simulink model "zhengji"  (Simulink 8.3)
settings: Solver=ode45  StartTime=0.0  StopTime=100  RelTol=1e-3
libraries: simulink_need_slupdate x2
(part 3 of 3)

== system zhengji/GT2/LC/Subsystem3 ==
  Gz : Inport
  nz : Inport  Port=2
  Lookup Table (2-D) : Lookup2D  RowIndex=[4300 5000 5500 6000 6500 7000 7500 8000]  ColumnIndex=[20:0.5:100]  Table=|
      | [1.1111 1.1471 1.1832 1.2192 1.2552 1.2913 1.3273 1.3633 1.3994 1.4354 1.4714 1.5074 1.5435 1.5795 1.6155 1.6516 1.6876 1.7236 1.8750 1.8749 1.8720 1.8623 1.8457 1.8223 1.7920 1.7549 1.7109 1.6601 1.6024 1.5378 1.4664 1.3881 1.2420 1.2701 1.2983 1.3265 1.3547 1.3828 1.4110 1.4392 1.4673 1.4955 1.5237 1.5519 1.5800 1.6082 1.6364 1.6645 1.6927 1.7209 1.7491 1.7772 1.8054 1.8336 1.8617 1.8899 1.9181 1.9463 1.9744 2.0026 2.0308 2.0590 2.0871 2.1153 2.1435 2.1716 2.1998 2.2280 2.2562 2.2843 2.3125 2.3407 2.3688 2.3970 2.4252 2.4534 2.4815 2.5097 2.5379 2.5660 2.5942 2.6224 2.6506 2.6787 2.7069 2.7351 2.7633 2.7914 2.8196 2.8478 2.8759 2.9041 2.9323 2.9605 2.9886 3.0168 3.0450 3.0731 3.1013 3.1295 3.1577 3.1858 3.2140 3.2422 3.2703 3.2985 3.3267 3.3549 3.3830 3.4112 3.4394 3.4676 3.4957 3.5239 3.5521 3.5802 3.6084 3.6366 3.6648 3.6929 3.7211 3.7493 3.7774 3.8056 3.8338 3.8620 3.8901 3.9183 3.9465 3.9746 4.0028 4.0310 4.0592 4.0873 4.1155 4.1437 4.1719 4.2000 4.2282 4.2564 4.2845 4.3127 4.3409 4.3691 4.3972 4.4254 4.4536 4.4817 4.5099 4.5381 4.5663 4.5944 4.6226 4.6508 4.6789 4.7071 4.7353 4.7635 4.7916 4.8198 4.8480;
      | 1.1111 1.1471 1.1832 1.2192 1.2552 1.2913 1.3273 1.3633 1.3994 1.4354 1.4714 1.5074 1.5435 1.5795 1.6155 1.6516 1.6876 1.7236 1.7597 1.7957 1.8317 1.8678 1.9038 1.9398 1.9758 2.0119 2.0479 2.0839 2.1200 2.1560 2.1920 2.2281 2.2641 2.3001 2.3361 2.3722 2.4082 2.4442 2.4803 2.5163 2.5523 2.5884 2.5200 2.4780 2.3700 2.2800 2.1500 1.8820 1.6080 1.7209 1.7491 1.7772 1.8054 1.8336 1.8617 1.8899 1.9181 1.9463 1.9744 2.0026 2.0308 2.0590 2.0871 2.1153 2.1435 2.1716 2.1998 2.2280 2.2562 2.2843 2.3125 2.3407 2.3688 2.3970 2.4252 2.4534 2.4815 2.5097 2.5379 2.5660 2.5942 2.6224 2.6506 2.6787 2.7069 2.7351 2.7633 2.7914 2.8196 2.8478 2.8759 2.9041 2.9323 2.9605 2.9886 3.0168 3.0450 3.0731 3.1013 3.1295 3.1577 3.1858 3.2140 3.2422 3.2703 3.2985 3.3267 3.3549 3.3830 3.4112 3.4394 3.4676 3.4957 3.5239 3.5521 3.5802 3.6084 3.6366 3.6648 3.6929 3.7211 3.7493 3.7774 3.8056 3.8338 3.8620 3.8901 3.9183 3.9465 3.9746 4.0028 4.0310 4.0592 4.0873 4.1155 4.1437 4.1719 4.2000 4.2282 4.2564 4.2845 4.3127 4.3409 4.3691 4.3972 4.4254 4.4536 4.4817 4.5099 4.5381 4.5663 4.5944 4.6226 4.6508 4.6789 4.7071 4.7353 4.7635 4.7916 4.8198 4.8480;
      | 1.1111 1.1471 1.1832 1.2192 1.2552 1.2913 1.3273 1.3633 1.3994 1.4354 1.4714 1.5074 1.5435 1.5795 1.6155 1.6516 1.6876 1.7236 1.7597 1.7957 1.8317 1.8678 1.9038 1.9398 1.9758 2.0119 2.0479 2.0839 2.1200 2.1560 2.1920 2.2281 2.2641 2.3001 2.3361 2.3722 2.4082 2.4442 2.4803 2.5163 2.5523 2.5884 2.6244 2.6604 2.6965 2.7325 2.7685 2.8045 2.8406 2.8766 2.9126 2.9487 2.9847 3.0207 2.8905 2.8292 2.7444 2.6661 2.5443 2.4489 2.3700 2.1776 2.0217 2.1153 2.1435 2.1716 2.1998 2.2280 2.2562 2.2843 2.3125 2.3407 2.3688 2.3970 2.4252 2.4534 2.4815 2.5097 2.5379 2.5660 2.5942 2.6224 2.6506 2.6787 2.7069 2.7351 2.7633 2.7914 2.8196 2.8478 2.8759 2.9041 2.9323 2.9605 2.9886 3.0168 3.0450 3.0731 3.1013 3.1295 3.1577 3.1858 3.2140 3.2422 3.2703 3.2985 3.3267 3.3549 3.3830 3.4112 3.4394 3.4676 3.4957 3.5239 3.5521 3.5802 3.6084 3.6366 3.6648 3.6929 3.7211 3.7493 3.7774 3.8056 3.8338 3.8620 3.8901 3.9183 3.9465 3.9746 4.0028 4.0310 4.0592 4.0873 4.1155 4.1437 4.1719 4.2000 4.2282 4.2564 4.2845 4.3127 4.3409 4.3691 4.3972 4.4254 4.4536 4.4817 4.5099 4.5381 4.5663 4.5944 4.6226 4.6508 4.6789 4.7071 4.7353 4.7635 4.7916 4.8198 4.8480;
      | 1.1111 1.1471 1.1832 1.2192 1.2552 1.2913 1.3273 1.3633 1.3994 1.4354 1.4714 1.5074 1.5435 1.5795 1.6155 1.6516 1.6876 1.7236 1.7597 1.7957 1.8317 1.8678 1.9038 1.9398 1.9758 2.0119 2.0479 2.0839 2.1200 2.1560 2.1920 2.2281 2.2641 2.3001 2.3361 2.3722 2.4082 2.4442 2.4803 2.5163 2.5523 2.5884 2.6244 2.6604 2.6965 2.7325 2.7685 2.8045 2.8406 2.8766 2.9126 2.9487 2.9847 3.0207 3.0568 3.0928 3.1288 3.1648 3.2009 3.2369 3.2729 3.3090 3.3450 3.3810 3.3655 3.3396 3.3040 3.2587 3.2037 3.1389 3.0645 2.9803 2.8865 2.7829 2.6696 2.5466 2.4815 2.5097 2.5379 2.5660 2.5942 2.6224 2.6506 2.6787 2.7069 2.7351 2.7633 2.7914 2.8196 2.8478 2.8759 2.9041 2.9323 2.9605 2.9886 3.0168 3.0450 3.0731 3.1013 3.1295 3.1577 3.1858 3.2140 3.2422 3.2703 3.2985 3.3267 3.3549 3.3830 3.4112 3.4394 3.4676 3.4957 3.5239 3.5521 3.5802 3.6084 3.6366 3.6648 3.6929 3.7211 3.7493 3.7774 3.8056 3.8338 3.8620 3.8901 3.9183 3.9465 3.9746 4.0028 4.0310 4.0592 4.0873 4.1155 4.1437 4.1719 4.2000 4.2282 4.2564 4.2845 4.3127 4.3409 4.3691 4.3972 4.4254 4.4536 4.4817 4.5099 4.5381 4.5663 4.5944 4.6226 4.6508 4.6789 4.7071 4.7353 4.7635 4.7916 4.8198 4.8480;
      | 1.1111 1.1471 1.1832 1.2192 1.2552 1.2913 1.3273 1.3633 1.3994 1.4354 1.4714 1.5074 1.5435 1.5795 1.6155 1.6516 1.6876 1.7236 1.7597 1.7957 1.8317 1.8678 1.9038 1.9398 1.9758 2.0119 2.0479 2.0839 2.1200 2.1560 2.1920 2.2281 2.2641 2.3001 2.3361 2.3722 2.4082 2.4442 2.4803 2.5163 2.5523 2.5884 2.6244 2.6604 2.6965 2.7325 2.7685 2.8045 2.8406 2.8766 2.9126 2.9487 2.9847 3.0207 3.0568 3.0928 3.1288 3.1648 3.2009 3.2369 3.2729 3.3090 3.3450 3.3810 3.4171 3.4531 3.4891 3.5252 3.5612 3.5972 3.6332 3.6693 3.7053 3.7413 3.7774 3.8134 3.8494 3.8855 3.9215 3.9575 3.9936 4.0296 4.0656 4.1016 4.1377 4.1737 4.2097 4.2458 4.2818 4.3178 4.3646 4.3478 4.3218 4.2866 4.2421 4.1884 4.1254 4.0533 3.9718 3.8812 3.7813 3.6722 3.5538 3.4262 3.2894 3.2985 3.3267 3.3549 3.3830 3.4112 3.4394 3.4676 3.4957 3.5239 3.5521 3.5802 3.6084 3.6366 3.6648 3.6929 3.7211 3.7493 3.7774 3.8056 3.8338 3.8620 3.8901 3.9183 3.9465 3.9746 4.0028 4.0310 4.0592 4.0873 4.1155 4.1437 4.1719 4.2000 4.2282 4.2564 4.2845 4.3127 4.3409 4.3691 4.3972 4.4254 4.4536 4.4817 4.5099 4.5381 4.5663 4.5944 4.6226 4.6508 4.6789 4.7071 4.7353 4.7635 4.7916 4.8198 4.8480;
      | 1.1111 1.1471 1.1832 1.2192 1.2552 1.2913 1.3273 1.3633 1.3994 1.4354 1.4714 1.5074 1.5435 1.5795 1.6155 1.6516 1.6876 1.7236 1.7597 1.7957 1.8317 1.8678 1.9038 1.9398 1.9758 2.0119 2.0479 2.0839 2.1200 2.1560 2.1920 2.2281 2.2641 2.3001 2.3361 2.3722 2.4082 2.4442 2.4803 2.5163 2.5523 2.5884 2.6244 2.6604 2.6965 2.7325 2.7685 2.8045 2.8406 2.8766 2.9126 2.9487 2.9847 3.0207 3.0568 3.0928 3.1288 3.1648 3.2009 3.2369 3.2729 3.3090 3.3450 3.3810 3.4171 3.4531 3.4891 3.5252 3.5612 3.5972 3.6332 3.6693 3.7053 3.7413 3.7774 3.8134 3.8494 3.8855 3.9215 3.9575 3.9936 4.0296 4.0656 4.1016 4.1377 4.1737 4.2097 4.2458 4.2818 4.3178 4.3539 4.3899 4.4259 4.4619 4.4980 4.5340 4.5700 4.6061 4.6421 4.6781 4.7142 4.7502 4.7862 4.8223 4.8583 4.8943 4.9303 4.9664 5.0024 5.0384 5.0745 5.1105 5.1465 5.3241 5.3091 5.2474 5.1391 4.9841 4.7824 4.5341 4.2392 3.8976 3.7774 3.8056 3.8338 3.8620 3.8901 3.9183 3.9465 3.9746 4.0028 4.0310 4.0592 4.0873 4.1155 4.1437 4.1719 4.2000 4.2282 4.2564 4.2845 4.3127 4.3409 4.3691 4.3972 4.4254 4.4536 4.4817 4.5099 4.5381 4.5663 4.5944 4.6226 4.6508 4.6789 4.7071 4.7353 4.7635 4.7916 4.8198 4.8480;
      | 1.1111 1.1471 1.1832 1.2192 1.2552 1.2913 1.3273 1.3633 1.3994 1.4354 1.4714 1.5074 1.5435 1.5795 1.6155 1.6516 1.6876 1.7236 1.7597 1.7957 1.8317 1.8678 1.9038 1.9398 1.9758 2.0119 2.0479 2.0839 2.1200 2.1560 2.1920 2.2281 2.2641 2.3001 2.3361 2.3722 2.4082 2.4442 2.4803 2.5163 2.5523 2.5884 2.6244 2.6604 2.6965 2.7325 2.7685 2.8045 2.8406 2.8766 2.9126 2.9487 2.9847 3.0207 3.0568 3.0928 3.1288 3.1648 3.2009 3.2369 3.2729 3.3090 3.3450 3.3810 3.4171 3.4531 3.4891 3.5252 3.5612 3.5972 3.6332 3.6693 3.7053 3.7413 3.7774 3.8134 3.8494 3.8855 3.9215 3.9575 3.9936 4.0296 4.0656 4.1016 4.1377 4.1737 4.2097 4.2458 4.2818 4.3178 4.3539 4.3899 4.4259 4.4619 4.4980 4.5340 4.5700 4.6061 4.6421 4.6781 4.7142 4.7502 4.7862 4.8223 4.8583 4.8943 4.9303 4.9664 5.0024 5.0384 5.0745 5.1105 5.1465 5.1826 5.2186 5.2546 5.2906 5.3267 5.3627 5.3987 5.4348 5.4708 5.5068 5.5429 5.5789 5.6149 5.6510 5.6870 5.7230 5.7590 5.7951 5.8311 5.8671 5.9032 5.9392 5.9752 6.0113 6.0473 5.2600 4.2400 4.2845 4.3127 4.3409 4.3691 4.3972 4.4254 4.4536 4.4817 4.5099 4.5381 4.5663 4.5944 4.6226 4.6508 4.6789 4.7071 4.7353 4.7635 4.7916 4.8198 4.8480;
      | 1.1111 1.1471 1.1832 1.2192 1.2552 1.2913 1.3273 1.3633 1.3994 1.4354 1.4714 1.5074 1.5435 1.5795 1.6155 1.6516 1.6876 1.7236 1.7597 1.7957 1.8317 1.8678 1.9038 1.9398 1.9758 2.0119 2.0479 2.0839 2.1200 2.1560 2.1920 2.2281 2.2641 2.3001 2.3361 2.3722 2.4082 2.4442 2.4803 2.5163 2.5523 2.5884 2.6244 2.6604 2.6965 2.7325 2.7685 2.8045 2.8406 2.8766 2.9126 2.9487 2.9847 3.0207 3.0568 3.0928 3.1288 3.1648 3.2009 3.2369 3.2729 3.3090 3.3450 3.3810 3.4171 3.4531 3.4891 3.5252 3.5612 3.5972 3.6332 3.6693 3.7053 3.7413 3.7774 3.8134 3.8494 3.8855 3.9215 3.9575 3.9936 4.0296 4.0656 4.1016 4.1377 4.1737 4.2097 4.2458 4.2818 4.3178 4.3539 4.3899 4.4259 4.4619 4.4980 4.5340 4.5700 4.6061 4.6421 4.6781 4.7142 4.7502 4.7862 4.8223 4.8583 4.8943 4.9303 4.9664 5.0024 5.0384 5.0745 5.1105 5.1465 5.1826 5.2186 5.2546 5.2906 5.3267 5.3627 5.3987 5.4348 5.4708 5.5068 5.5429 5.5789 5.6149 5.6510 5.6870 5.7230 5.7590 5.7951 5.8311 5.8671 5.9032 5.9392 5.9752 6.0113 6.0473 6.0833 6.1193 6.1554 6.1914 6.2274 6.2635 6.2995 6.3355 6.3716 6.4076 6.4436 6.4797 6.5157 6.5517 6.5877 6.6238 6.6598 4.7071 4.7353 4.7635 4.7916 4.8198 4.8480;]
  Lookup Table (2-D)1 : Lookup2D  RowIndex=[4300 5000 5500 6000 6500 7000 7500 8000]  ColumnIndex=[20:0.5:100]  Table=|
      | [0.8303 0.8307 0.8310 0.8314 0.8317 0.8321 0.8324 0.8327 0.8331 0.8335 0.8338 0.8341 0.8345 0.8348 0.8351 0.8355 0.8358 0.8361 0.8371 0.8390 0.8403 0.8412 0.8415 0.8412 0.8405 0.8392 0.8373 0.8350 0.8321 0.8287 0.8247 0.8203 0.8200 0.8200 0.8200 0.8200 0.8200 0.8200 0.8200 0.8200 0.8200 0.8200 0.8200 0.8200 0.8200 0.8200 0.8200 0.8200 0.8200 0.8200 0.8200 0.8200 0.8200 0.8200 0.8200 0.8200 0.8200 0.8200 0.8200 0.8200 0.8200 0.8200 0.8200 0.8200 0.8200 0.8200 0.8200 0.8200 0.8200 0.8200 0.8200 0.8200 0.8200 0.8200 0.8200 0.8200 0.8200 0.8200 0.8200 0.8200 0.8200 0.8200 0.8200 0.8200 0.8200 0.8200 0.8200 0.8200 0.8200 0.8200 0.8200 0.8200 0.8200 0.8200 0.8200 0.8200 0.8200 0.8200 0.8200 0.8200 0.8200 0.8200 0.8200 0.8200 0.8200 0.8500 0.8500 0.8500 0.8500 0.8500 0.8500 0.8500 0.8500 0.8500 0.8500 0.8500 0.8500 0.8500 0.8500 0.8500 0.8500 0.8500 0.8500 0.8500 0.8500 0.8500 0.8500 0.8500 0.8500 0.8500 0.8500 0.8500 0.8500 0.8500 0.8500 0.8500 0.8500 0.8500 0.8500 0.8500 0.8500 0.8500 0.8500 0.8500 0.8500 0.8500 0.8500 0.8500 0.8500 0.8500 0.8500 0.8500 0.8500 0.8500 0.8500 0.8500 0.8500 0.8500 0.8500 0.8500 0.8500;
      | 0.8303 0.8307 0.8310 0.8314 0.8317 0.8321 0.8324 0.8327 0.8331 0.8335 0.8338 0.8341 0.8345 0.8348 0.8351 0.8355 0.8358 0.8361 0.8371 0.8375 0.8379 0.8383 0.8387 0.8391 0.8395 0.8400 0.8402 0.8405 0.8407 0.8410 0.8412 0.8415 0.8417 0.8420 0.8422 0.8425 0.8427 0.8430 0.8432 0.8435 0.8437 0.8440 0.8441 0.8727 0.8851 0.8814 0.8616 0.8257 0.8200 0.8200 0.8200 0.8200 0.8200 0.8200 0.8200 0.8200 0.8200 0.8200 0.8200 0.8200 0.8200 0.8200 0.8200 0.8200 0.8200 0.8200 0.8200 0.8200 0.8200 0.8200 0.8200 0.8200 0.8200 0.8200 0.8200 0.8200 0.8200 0.8200 0.8200 0.8200 0.8200 0.8200 0.8200 0.8200 0.8200 0.8200 0.8200 0.8200 0.8200 0.8200 0.8200 0.8200 0.8200 0.8200 0.8200 0.8200 0.8200 0.8200 0.8200 0.8200 0.8200 0.8200 0.8200 0.8200 0.8200 0.8500 0.8500 0.8500 0.8500 0.8500 0.8500 0.8500 0.8500 0.8500 0.8500 0.8500 0.8500 0.8500 0.8500 0.8500 0.8500 0.8500 0.8500 0.8500 0.8500 0.8500 0.8500 0.8500 0.8500 0.8500 0.8500 0.8500 0.8500 0.8500 0.8500 0.8500 0.8500 0.8500 0.8500 0.8500 0.8500 0.8500 0.8500 0.8500 0.8500 0.8500 0.8500 0.8500 0.8500 0.8500 0.8500 0.8500 0.8500 0.8500 0.8500 0.8500 0.8500 0.8500 0.8500 0.8500 0.8500;
      | 0.8303 0.8307 0.8310 0.8314 0.8317 0.8321 0.8324 0.8327 0.8331 0.8335 0.8338 0.8341 0.8345 0.8348 0.8351 0.8355 0.8358 0.8361 0.8371 0.8375 0.8379 0.8383 0.8387 0.8391 0.8395 0.8400 0.8402 0.8405 0.8407 0.8410 0.8412 0.8415 0.8417 0.8420 0.8422 0.8425 0.8427 0.8430 0.8432 0.8435 0.8437 0.8440 0.8441 0.8440 0.8440 0.8440 0.8440 0.8440 0.8400 0.8400 0.8400 0.8400 0.8400 0.8400 0.8400 0.8400 0.8420 0.8439 0.8592 0.8652 0.8619 0.8495 0.8278 0.8200 0.8200 0.8200 0.8200 0.8200 0.8200 0.8200 0.8200 0.8200 0.8200 0.8200 0.8200 0.8200 0.8200 0.8200 0.8200 0.8200 0.8200 0.8200 0.8200 0.8200 0.8200 0.8200 0.8200 0.8200 0.8200 0.8200 0.8200 0.8200 0.8200 0.8200 0.8200 0.8200 0.8200 0.8200 0.8200 0.8200 0.8200 0.8200 0.8200 0.8200 0.8200 0.8500 0.8500 0.8500 0.8500 0.8500 0.8500 0.8500 0.8500 0.8500 0.8500 0.8500 0.8500 0.8500 0.8500 0.8500 0.8500 0.8500 0.8500 0.8500 0.8500 0.8500 0.8500 0.8500 0.8500 0.8500 0.8500 0.8500 0.8500 0.8500 0.8500 0.8500 0.8500 0.8500 0.8500 0.8500 0.8500 0.8500 0.8500 0.8500 0.8500 0.8500 0.8500 0.8500 0.8500 0.8500 0.8500 0.8500 0.8500 0.8500 0.8500 0.8500 0.8500 0.8500 0.8500 0.8500 0.8500;
      | 0.8303 0.8307 0.8310 0.8314 0.8317 0.8321 0.8324 0.8327 0.8331 0.8335 0.8338 0.8341 0.8345 0.8348 0.8351 0.8355 0.8358 0.8361 0.8371 0.8375 0.8379 0.8383 0.8387 0.8391 0.8395 0.8400 0.8402 0.8405 0.8407 0.8410 0.8412 0.8415 0.8417 0.8420 0.8422 0.8425 0.8427 0.8430 0.8432 0.8435 0.8437 0.8440 0.8441 0.8440 0.8440 0.8440 0.8440 0.8440 0.8400 0.8400 0.8400 0.8400 0.8400 0.8400 0.8400 0.8390 0.8380 0.8370 0.8360 0.8350 0.8340 0.8330 0.8320 0.8310 0.8300 0.8300 0.8300 0.8371 0.8489 0.8568 0.8608 0.8609 0.8570 0.8492 0.8375 0.8219 0.8200 0.8200 0.8200 0.8200 0.8200 0.8200 0.8200 0.8200 0.8200 0.8200 0.8200 0.8200 0.8200 0.8200 0.8200 0.8200 0.8200 0.8200 0.8200 0.8200 0.8200 0.8200 0.8200 0.8200 0.8200 0.8200 0.8200 0.8200 0.8200 0.8500 0.8500 0.8500 0.8500 0.8500 0.8500 0.8500 0.8500 0.8500 0.8500 0.8500 0.8500 0.8500 0.8500 0.8500 0.8500 0.8500 0.8500 0.8500 0.8500 0.8500 0.8500 0.8500 0.8500 0.8500 0.8500 0.8500 0.8500 0.8500 0.8500 0.8500 0.8500 0.8500 0.8500 0.8500 0.8500 0.8500 0.8500 0.8500 0.8500 0.8500 0.8500 0.8500 0.8500 0.8500 0.8500 0.8500 0.8500 0.8500 0.8500 0.8500 0.8500 0.8500 0.8500 0.8500 0.8500;
      | 0.8303 0.8307 0.8310 0.8314 0.8317 0.8321 0.8324 0.8327 0.8331 0.8335 0.8338 0.8341 0.8345 0.8348 0.8351 0.8355 0.8358 0.8361 0.8371 0.8375 0.8379 0.8383 0.8387 0.8391 0.8395 0.8400 0.8402 0.8405 0.8407 0.8410 0.8412 0.8415 0.8417 0.8420 0.8422 0.8425 0.8427 0.8430 0.8432 0.8435 0.8437 0.8440 0.8441 0.8440 0.8440 0.8440 0.8440 0.8440 0.8400 0.8400 0.8400 0.8400 0.8400 0.8400 0.8400 0.8390 0.8380 0.8370 0.8360 0.8350 0.8340 0.8330 0.8320 0.8310 0.8300 0.8306 0.8312 0.8318 0.8324 0.8330 0.8336 0.8342 0.8348 0.8354 0.8360 0.8366 0.8372 0.8378 0.8384 0.8390 0.8396 0.8402 0.8408 0.8414 0.8420 0.8426 0.8432 0.8435 0.8438 0.8442 0.8438 0.8515 0.8581 0.8636 0.8680 0.8712 0.8733 0.8743 0.8742 0.8730 0.8706 0.8671 0.8625 0.8568 0.8500 0.8500 0.8500 0.8500 0.8500 0.8500 0.8500 0.8500 0.8500 0.8500 0.8500 0.8500 0.8500 0.8500 0.8500 0.8500 0.8500 0.8500 0.8500 0.8500 0.8500 0.8500 0.8500 0.8500 0.8500 0.8500 0.8500 0.8500 0.8500 0.8500 0.8500 0.8500 0.8500 0.8500 0.8500 0.8500 0.8500 0.8500 0.8500 0.8500 0.8500 0.8500 0.8500 0.8500 0.8500 0.8500 0.8500 0.8500 0.8500 0.8500 0.8500 0.8500 0.8500 0.8500 0.8500 0.8500 0.8500;
      | 0.8303 0.8307 0.8310 0.8314 0.8317 0.8321 0.8324 0.8327 0.8331 0.8335 0.8338 0.8341 0.8345 0.8348 0.8351 0.8355 0.8358 0.8361 0.8371 0.8375 0.8379 0.8383 0.8387 0.8391 0.8395 0.8400 0.8402 0.8405 0.8407 0.8410 0.8412 0.8415 0.8417 0.8420 0.8422 0.8425 0.8427 0.8430 0.8432 0.8435 0.8437 0.8440 0.8441 0.8440 0.8440 0.8440 0.8440 0.8440 0.8400 0.8400 0.8400 0.8400 0.8400 0.8400 0.8400 0.8390 0.8380 0.8370 0.8360 0.8350 0.8340 0.8330 0.8320 0.8310 0.8300 0.8306 0.8312 0.8318 0.8324 0.8330 0.8336 0.8342 0.8348 0.8354 0.8360 0.8366 0.8372 0.8378 0.8384 0.8390 0.8396 0.8402 0.8408 0.8414 0.8420 0.8426 0.8432 0.8435 0.8438 0.8442 0.8448 0.8452 0.8457 0.8462 0.8467 0.8472 0.8476 0.8451 0.8486 0.8491 0.8496 0.8500 0.8505 0.8510 0.8515 0.8520 0.8524 0.8529 0.8534 0.8539 0.8544 0.8548 0.8549 0.8550 0.8600 0.8650 0.8746 0.8872 0.8921 0.8890 0.8782 0.8595 0.8500 0.8500 0.8500 0.8500 0.8500 0.8500 0.8500 0.8500 0.8500 0.8500 0.8500 0.8500 0.8500 0.8500 0.8500 0.8500 0.8500 0.8500 0.8500 0.8500 0.8500 0.8500 0.8500 0.8500 0.8500 0.8500 0.8500 0.8500 0.8500 0.8500 0.8500 0.8500 0.8500 0.8500 0.8500 0.8500 0.8500 0.8500 0.8500;
      | 0.8303 0.8307 0.8310 0.8314 0.8317 0.8321 0.8324 0.8327 0.8331 0.8335 0.8338 0.8341 0.8345 0.8348 0.8351 0.8355 0.8358 0.8361 0.8371 0.8375 0.8379 0.8383 0.8387 0.8391 0.8395 0.8400 0.8402 0.8405 0.8407 0.8410 0.8412 0.8415 0.8417 0.8420 0.8422 0.8425 0.8427 0.8430 0.8432 0.8435 0.8437 0.8440 0.8441 0.8440 0.8440 0.8440 0.8440 0.8440 0.8400 0.8400 0.8400 0.8400 0.8400 0.8400 0.8400 0.8390 0.8380 0.8370 0.8360 0.8350 0.8340 0.8330 0.8320 0.8310 0.8300 0.8306 0.8312 0.8318 0.8324 0.8330 0.8336 0.8342 0.8348 0.8354 0.8360 0.8366 0.8372 0.8378 0.8384 0.8390 0.8396 0.8402 0.8408 0.8414 0.8420 0.8426 0.8432 0.8435 0.8438 0.8442 0.8448 0.8452 0.8457 0.8462 0.8467 0.8472 0.8476 0.8451 0.8486 0.8491 0.8496 0.8500 0.8505 0.8510 0.8515 0.8520 0.8524 0.8529 0.8534 0.8539 0.8544 0.8548 0.8549 0.8550 0.8550 0.8550 0.8550 0.8550 0.8550 0.8550 0.8550 0.8550 0.8550 0.8550 0.8550 0.8550 0.8550 0.8550 0.8550 0.8550 0.8550 0.8550 0.8550 0.8550 0.8550 0.8550 0.8550 0.8550 0.8788 0.8500 0.8500 0.8500 0.8500 0.8500 0.8500 0.8500 0.8500 0.8500 0.8500 0.8500 0.8500 0.8500 0.8500 0.8500 0.8500 0.8500 0.8500 0.8500 0.8500 0.8500 0.8500;
      | 0.8303 0.8307 0.8310 0.8314 0.8317 0.8321 0.8324 0.8327 0.8331 0.8335 0.8338 0.8341 0.8345 0.8348 0.8351 0.8355 0.8358 0.8361 0.8371 0.8375 0.8379 0.8383 0.8387 0.8391 0.8395 0.8400 0.8402 0.8405 0.8407 0.8410 0.8412 0.8415 0.8417 0.8420 0.8422 0.8425 0.8427 0.8430 0.8432 0.8435 0.8437 0.8440 0.8441 0.8440 0.8440 0.8440 0.8440 0.8440 0.8400 0.8400 0.8400 0.8400 0.8400 0.8400 0.8400 0.8390 0.8380 0.8370 0.8360 0.8350 0.8340 0.8330 0.8320 0.8310 0.8300 0.8306 0.8312 0.8318 0.8324 0.8330 0.8336 0.8342 0.8348 0.8354 0.8360 0.8366 0.8372 0.8378 0.8384 0.8390 0.8396 0.8402 0.8408 0.8414 0.8420 0.8426 0.8432 0.8435 0.8438 0.8442 0.8448 0.8452 0.8457 0.8462 0.8467 0.8472 0.8476 0.8451 0.8486 0.8491 0.8496 0.8500 0.8505 0.8510 0.8515 0.8520 0.8524 0.8529 0.8534 0.8539 0.8544 0.8548 0.8549 0.8550 0.8550 0.8550 0.8550 0.8550 0.8550 0.8550 0.8550 0.8550 0.8550 0.8550 0.8550 0.8550 0.8550 0.8550 0.8550 0.8550 0.8550 0.8550 0.8550 0.8550 0.8550 0.8550 0.8550 0.8550 0.8550 0.8550 0.8550 0.8550 0.8550 0.8550 0.8550 0.8550 0.8550 0.8550 0.8550 0.8550 0.8550 0.8550 0.8550 0.8550 0.8550 0.8550 0.8500 0.8500 0.8500 0.8500 0.8550;]
  pi : Outport
  eta : Outport  Port=2
  wires:
  nz/1 -> Lookup Table (2-D)/1, Lookup Table (2-D)1/1
  Gz/1 -> Lookup Table (2-D)1/2, Lookup Table (2-D)/2
  Lookup Table (2-D)/1 -> pi/1
  Lookup Table (2-D)1/1 -> eta/1

== system zhengji/GT2/LC/compresser_TN ==
  Gin : Inport
  Pi : Inport  Port=2
  eta : Inport  Port=3
  Tin : Inport  Port=4
  Add : Sum  Inputs=+-
  Add1 : Sum
  Constant : Constant
  Divide : Product  Inputs=/*
  Fcn : Fcn  Expr=u[1]^(u[2])
  K : Subsystem
  K1 : Constant  Value=1.4
  Mux : Mux  Inputs=2
  Product : Product  Inputs=4  RndMeth=Zero
  Product1 : Product  RndMeth=Zero
  m : Fcn  Expr=(u-1)/u
  Tout : Outport
  Nout : Outport  Port=2
  wires:
  Tin/1 -> K/1(T1), Product1/2, Product/4
  Pi/1 -> Mux/1
  m/1 -> Mux/2
  Mux/1 -> Fcn/1
  Fcn/1 -> Add/1
  Add/1 -> Divide/2
  eta/1 -> Divide/1
  Divide/1 -> Add1/1, Product/1
  Constant/1 -> Add/2, Add1/2
  Product1/1 -> Tout/1
  Product/1 -> Nout/1
  Add1/1 -> Product1/1
  K/2(Cp) -> Product/2
  Gin/1 -> Product/3
  K1/1 -> m/1

== system zhengji/GT2/LC/zhehe ==
  n : Inport
  Tin : Inport  Port=2
  Divide : Product  Inputs=*/
  Fcn : Fcn  Expr=sqrt(u/288)
  nz : Outport
  wires:
  Tin/1 -> Fcn/1
  n/1 -> Divide/1
  Fcn/1 -> Divide/2
  Divide/1 -> nz/1

== system zhengji/GT2/LT/turbine_TN ==
  Pi : Inport
  eta : Inport  Port=2
  Tin : Inport  Port=3
  Gin : Inport  Port=4
  Add : Sum  Inputs=-+
  Add1 : Sum  Inputs=-+
  Constant : Constant
  Fcn : Fcn  Expr=1/(u[1]^u[2])
  K : Subsystem
  K1 : Constant  Value=1.33
  Mux : Mux  Inputs=2
  Product : Product  Inputs=4  RndMeth=Zero
  Product1 : Product  RndMeth=Zero
  Product2 : Product  RndMeth=Zero
  m : Fcn  Expr=(u-1)/u
  Tout : Outport
  Nout : Outport  Port=2
  wires:
  Tin/1 -> K/1(T1), Product1/2, Product/4
  Pi/1 -> Mux/1
  m/1 -> Mux/2
  Mux/1 -> Fcn/1
  Fcn/1 -> Add/1
  Add/1 -> Product2/2
  eta/1 -> Product2/1
  Product2/1 -> Add1/1, Product/1
  Constant/1 -> Add/2, Add1/2
  Product1/1 -> Tout/1
  Product/1 -> Nout/1
  Add1/1 -> Product1/1
  K/2(Cp) -> Product/2
  Gin/1 -> Product/3
  K1/1 -> m/1

== system zhengji/GT2/PT/turbine_TN ==
  Pi : Inport
  eta : Inport  Port=2
  Gin : Inport  Port=3
  Tin : Inport  Port=4
  Add : Sum  Inputs=-+
  Add1 : Sum  Inputs=-+
  Constant : Constant
  Fcn : Fcn  Expr=1/(u[1]^u[2])
  K1 : Subsystem
  Mux : Mux  Inputs=2
  Product : Product  Inputs=4  RndMeth=Zero
  Product1 : Product  RndMeth=Zero
  Product2 : Product  RndMeth=Zero
  m : Fcn  Expr=(u-1)/u
  Tout : Outport
  Nout : Outport  Port=2
  wires:
  Pi/1 -> Mux/1
  m/1 -> Mux/2
  Mux/1 -> Fcn/1
  Fcn/1 -> Add/1
  Add/1 -> Product2/2
  eta/1 -> Product2/1
  Product2/1 -> Add1/1, Product/1
  Constant/1 -> Add/2, Add1/2
  Product1/1 -> Tout/1
  Product/1 -> Nout/1
  Add1/1 -> Product1/1
  Gin/1 -> Product/3
  Tin/1 -> K1/1(T1), Product1/2, Product/4
  K1/2(Cp) -> Product/2
  K1/1(K) -> m/1

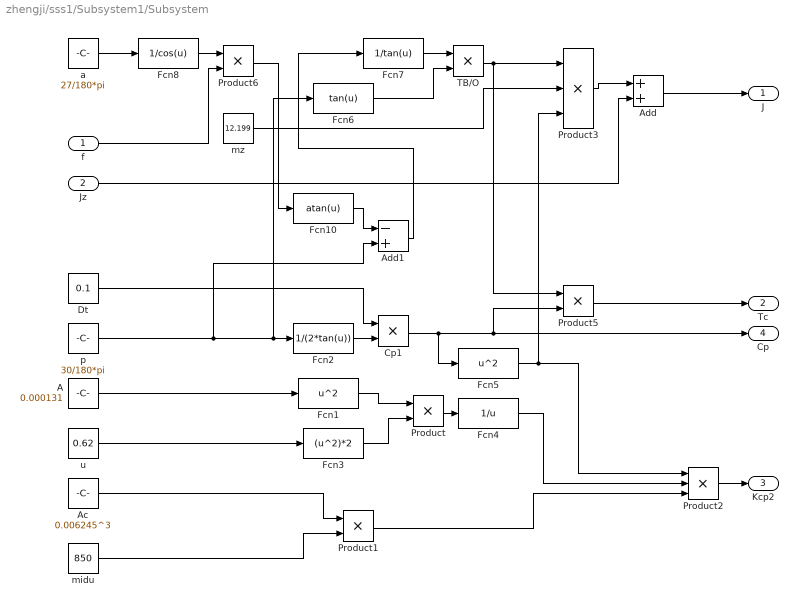
== system zhengji/sss1/Subsystem1/Subsystem ==
  f : Inport
  Jz : Inport  Port=2
  A : Constant  Value=0.000131
  Ac : Constant  Value=0.006245^3
  Add : Sum
  Add1 : Sum  Inputs=-+
  Cp1 : Product  RndMeth=Zero
  Dt : Constant  Value=0.1
  Fcn1 : Fcn  Expr=u^2
  Fcn10 : Fcn  Expr=atan(u)
  Fcn2 : Fcn  Expr=1/(2*tan(u))
  Fcn3 : Fcn  Expr=(u^2)*2
  Fcn4 : Fcn  Expr=1/u
  Fcn5 : Fcn  Expr=u^2
  Fcn6 : Fcn  Expr=tan(u)
  Fcn7 : Fcn  Expr=1/tan(u)
  Fcn8 : Fcn  Expr=1/cos(u)
  Product{,1,5..6} (4 alike) : Product  RndMeth=Zero
  Product2 : Product  Inputs=3  RndMeth=Zero
  Product3 : Product  Inputs=3  RndMeth=Zero
  TB/O : Product  RndMeth=Zero
  a : Constant  Value=27/180*pi
  midu : Constant  Value=850
  mz : Constant  Value=12.199
  p : Constant  Value=30/180*pi
  u : Constant  Value=0.62
  J : Outport
  Tc : Outport  Port=2
  Kcp2 : Outport  Port=3
  Cp : Outport  Port=4
  wires:
  p/1 -> Fcn2/1, Fcn6/1, Add1/2
  Dt/1 -> Cp1/1
  Fcn2/1 -> Cp1/2
  Cp1/1 -> Cp/1, Product5/2, Fcn5/1
  A/1 -> Fcn1/1
  u/1 -> Fcn3/1
  Fcn3/1 -> Product/2
  Fcn1/1 -> Product/1
  Product/1 -> Fcn4/1
  Ac/1 -> Product1/1
  midu/1 -> Product1/2
  Product1/1 -> Product2/3
  Product2/1 -> Kcp2/1
  Fcn4/1 -> Product2/2
  Fcn5/1 -> Product2/1, Product3/3
  a/1 -> Fcn8/1
  Product3/1 -> Add/1
  Jz/1 -> Add/2
  Add/1 -> J/1
  Fcn7/1 -> TB/O/1
  Fcn6/1 -> TB/O/2
  TB/O/1 -> Product3/1, Product5/1
  mz/1 -> Product3/2
  Product5/1 -> Tc/1
  Fcn8/1 -> Product6/1
  f/1 -> Product6/2
  Product6/1 -> Fcn10/1
  Fcn10/1 -> Add1/1
  Add1/1 -> Fcn7/1

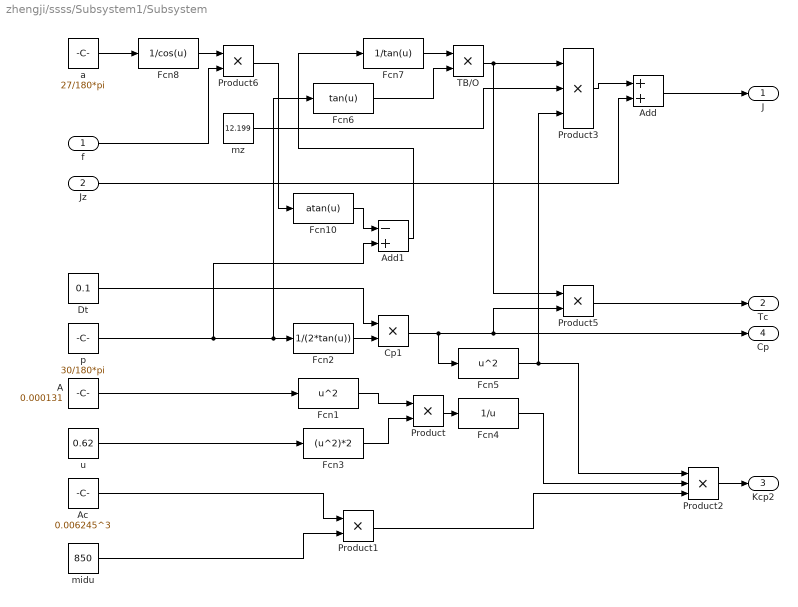
== system zhengji/ssss/Subsystem1/Subsystem ==
  f : Inport
  Jz : Inport  Port=2
  A : Constant  Value=0.000131
  Ac : Constant  Value=0.006245^3
  Add : Sum
  Add1 : Sum  Inputs=-+
  Cp1 : Product  RndMeth=Zero
  Dt : Constant  Value=0.1
  Fcn1 : Fcn  Expr=u^2
  Fcn10 : Fcn  Expr=atan(u)
  Fcn2 : Fcn  Expr=1/(2*tan(u))
  Fcn3 : Fcn  Expr=(u^2)*2
  Fcn4 : Fcn  Expr=1/u
  Fcn5 : Fcn  Expr=u^2
  Fcn6 : Fcn  Expr=tan(u)
  Fcn7 : Fcn  Expr=1/tan(u)
  Fcn8 : Fcn  Expr=1/cos(u)
  Product{,1,5..6} (4 alike) : Product  RndMeth=Zero
  Product2 : Product  Inputs=3  RndMeth=Zero
  Product3 : Product  Inputs=3  RndMeth=Zero
  TB/O : Product  RndMeth=Zero
  a : Constant  Value=27/180*pi
  midu : Constant  Value=850
  mz : Constant  Value=12.199
  p : Constant  Value=30/180*pi
  u : Constant  Value=0.62
  J : Outport
  Tc : Outport  Port=2
  Kcp2 : Outport  Port=3
  Cp : Outport  Port=4
  wires:
  p/1 -> Fcn2/1, Fcn6/1, Add1/2
  Dt/1 -> Cp1/1
  Fcn2/1 -> Cp1/2
  Cp1/1 -> Cp/1, Product5/2, Fcn5/1
  A/1 -> Fcn1/1
  u/1 -> Fcn3/1
  Fcn3/1 -> Product/2
  Fcn1/1 -> Product/1
  Product/1 -> Fcn4/1
  Ac/1 -> Product1/1
  midu/1 -> Product1/2
  Product1/1 -> Product2/3
  Product2/1 -> Kcp2/1
  Fcn4/1 -> Product2/2
  Fcn5/1 -> Product2/1, Product3/3
  a/1 -> Fcn8/1
  Product3/1 -> Add/1
  Jz/1 -> Add/2
  Add/1 -> J/1
  Fcn7/1 -> TB/O/1
  Fcn6/1 -> TB/O/2
  TB/O/1 -> Product3/1, Product5/1
  mz/1 -> Product3/2
  Product5/1 -> Tc/1
  Fcn8/1 -> Product6/1
  f/1 -> Product6/2
  Product6/1 -> Fcn10/1
  Fcn10/1 -> Add1/1
  Add1/1 -> Fcn7/1

== system zhengji/GT1/HC/compresser_TN/K ==
  note: Cv
  note: Cp
  T1 : Inport
  Add : Sum
  Add1 : Sum
  Add2 : Sum  Inputs=+-
  Constant : Constant  Value=0.9956
  Constant1 : Constant  Value=0.7088
  Divide1 : Product  Inputs=*/
  Gain2 : Gain  Gain=0.000093
  Gain3 : Gain  Gain=0.000093
  Scope3 : Scope
      settings: YMin=2829.54  YMax=3127.38  SaveName=ScopeData23
  Tk : Constant  Value=273.15
  K : Outport
  Cp : Outport  Port=2
  wires:
  Divide1/1 -> K/1, Scope3/1
  Add1/1 -> Divide1/2
  Constant1/1 -> Add1/2
  Gain3/1 -> Add1/1
  Add/1 -> Divide1/1, Cp/1
  Constant/1 -> Add/2
  Gain2/1 -> Add/1
  T1/1 -> Add2/1
  Tk/1 -> Add2/2
  Add2/1 -> Gain2/1, Gain3/1

== system zhengji/GT1/HT/turbine_TN/K ==
  note: Cv
  note: Cp
  T1 : Inport
  Add : Sum
  Add1 : Sum
  Add2 : Sum  Inputs=+-
  Constant : Constant  Value=0.9956
  Constant1 : Constant  Value=0.7088
  Divide1 : Product  Inputs=*/
  Gain2 : Gain  Gain=0.000093
  Gain3 : Gain  Gain=0.000093
  Tk : Constant  Value=273.15
  K : Outport
  Cp : Outport  Port=2
  wires:
  Divide1/1 -> K/1
  Add1/1 -> Divide1/2
  Constant1/1 -> Add1/2
  Gain3/1 -> Add1/1
  Add/1 -> Divide1/1, Cp/1
  Constant/1 -> Add/2
  Gain2/1 -> Add/1
  T1/1 -> Add2/1
  Tk/1 -> Add2/2
  Add2/1 -> Gain2/1, Gain3/1

== system zhengji/GT1/LC/compresser_TN/K ==
  note: Cv
  note: Cp
  T1 : Inport
  Add : Sum
  Add1 : Sum
  Add2 : Sum  Inputs=+-
  Constant : Constant  Value=0.9956
  Constant1 : Constant  Value=0.7088
  Divide1 : Product  Inputs=*/
  Gain2 : Gain  Gain=0.000093
  Gain3 : Gain  Gain=0.000093
  Tk : Constant  Value=273.15
  K : Outport
  Cp : Outport  Port=2
  wires:
  Divide1/1 -> K/1
  Add1/1 -> Divide1/2
  Constant1/1 -> Add1/2
  Gain3/1 -> Add1/1
  Add/1 -> Divide1/1, Cp/1
  Constant/1 -> Add/2
  Gain2/1 -> Add/1
  T1/1 -> Add2/1
  Tk/1 -> Add2/2
  Add2/1 -> Gain2/1, Gain3/1

== system zhengji/GT1/LT/turbine_TN/K ==
  note: Cv
  note: Cp
  T1 : Inport
  Add : Sum
  Add1 : Sum
  Add2 : Sum  Inputs=+-
  Constant : Constant  Value=0.9956
  Constant1 : Constant  Value=0.7088
  Divide1 : Product  Inputs=*/
  Gain2 : Gain  Gain=0.000093
  Gain3 : Gain  Gain=0.000093
  Tk : Constant  Value=273.15
  K : Outport
  Cp : Outport  Port=2
  wires:
  Divide1/1 -> K/1
  Add1/1 -> Divide1/2
  Constant1/1 -> Add1/2
  Gain3/1 -> Add1/1
  Add/1 -> Divide1/1, Cp/1
  Constant/1 -> Add/2
  Gain2/1 -> Add/1
  T1/1 -> Add2/1
  Tk/1 -> Add2/2
  Add2/1 -> Gain2/1, Gain3/1

== system zhengji/GT1/PT/turbine_TN/K1 ==
  note: Cp
  note: Cv
  T1 : Inport
  Add : Sum
  Add1 : Sum
  Add2 : Sum  Inputs=+-
  Constant : Constant  Value=0.9956
  Constant1 : Constant  Value=0.7088
  Divide1 : Product  Inputs=*/
  Gain2 : Gain  Gain=0.000093
  Gain3 : Gain  Gain=0.000093
  Tk : Constant  Value=273.15
  K : Outport
  Cp : Outport  Port=2
  wires:
  Add/1 -> Divide1/1, Cp/1
  Constant/1 -> Add/2
  Gain2/1 -> Add/1
  T1/1 -> Add2/1
  Tk/1 -> Add2/2
  Add2/1 -> Gain2/1, Gain3/1
  Divide1/1 -> K/1
  Add1/1 -> Divide1/2
  Constant1/1 -> Add1/2
  Gain3/1 -> Add1/1

== system zhengji/GT2/HC/compresser_TN/K ==
  note: Cv
  note: Cp
  T1 : Inport
  Add : Sum
  Add1 : Sum
  Add2 : Sum  Inputs=+-
  Constant : Constant  Value=0.9956
  Constant1 : Constant  Value=0.7088
  Divide1 : Product  Inputs=*/
  Gain2 : Gain  Gain=0.000093
  Gain3 : Gain  Gain=0.000093
  Scope3 : Scope
      settings: YMin=2829.54  YMax=3127.38  SaveName=ScopeData23
  Tk : Constant  Value=273.15
  K : Outport
  Cp : Outport  Port=2
  wires:
  Divide1/1 -> K/1, Scope3/1
  Add1/1 -> Divide1/2
  Constant1/1 -> Add1/2
  Gain3/1 -> Add1/1
  Add/1 -> Divide1/1, Cp/1
  Constant/1 -> Add/2
  Gain2/1 -> Add/1
  T1/1 -> Add2/1
  Tk/1 -> Add2/2
  Add2/1 -> Gain2/1, Gain3/1

== system zhengji/GT2/HT/turbine_TN/K ==
  note: Cv
  note: Cp
  T1 : Inport
  Add : Sum
  Add1 : Sum
  Add2 : Sum  Inputs=+-
  Constant : Constant  Value=0.9956
  Constant1 : Constant  Value=0.7088
  Divide1 : Product  Inputs=*/
  Gain2 : Gain  Gain=0.000093
  Gain3 : Gain  Gain=0.000093
  Tk : Constant  Value=273.15
  K : Outport
  Cp : Outport  Port=2
  wires:
  Divide1/1 -> K/1
  Add1/1 -> Divide1/2
  Constant1/1 -> Add1/2
  Gain3/1 -> Add1/1
  Add/1 -> Divide1/1, Cp/1
  Constant/1 -> Add/2
  Gain2/1 -> Add/1
  T1/1 -> Add2/1
  Tk/1 -> Add2/2
  Add2/1 -> Gain2/1, Gain3/1

== system zhengji/GT2/LC/compresser_TN/K ==
  note: Cv
  note: Cp
  T1 : Inport
  Add : Sum
  Add1 : Sum
  Add2 : Sum  Inputs=+-
  Constant : Constant  Value=0.9956
  Constant1 : Constant  Value=0.7088
  Divide1 : Product  Inputs=*/
  Gain2 : Gain  Gain=0.000093
  Gain3 : Gain  Gain=0.000093
  Tk : Constant  Value=273.15
  K : Outport
  Cp : Outport  Port=2
  wires:
  Divide1/1 -> K/1
  Add1/1 -> Divide1/2
  Constant1/1 -> Add1/2
  Gain3/1 -> Add1/1
  Add/1 -> Divide1/1, Cp/1
  Constant/1 -> Add/2
  Gain2/1 -> Add/1
  T1/1 -> Add2/1
  Tk/1 -> Add2/2
  Add2/1 -> Gain2/1, Gain3/1

== system zhengji/GT2/LT/turbine_TN/K ==
  note: Cv
  note: Cp
  T1 : Inport
  Add : Sum
  Add1 : Sum
  Add2 : Sum  Inputs=+-
  Constant : Constant  Value=0.9956
  Constant1 : Constant  Value=0.7088
  Divide1 : Product  Inputs=*/
  Gain2 : Gain  Gain=0.000093
  Gain3 : Gain  Gain=0.000093
  Tk : Constant  Value=273.15
  K : Outport
  Cp : Outport  Port=2
  wires:
  Divide1/1 -> K/1
  Add1/1 -> Divide1/2
  Constant1/1 -> Add1/2
  Gain3/1 -> Add1/1
  Add/1 -> Divide1/1, Cp/1
  Constant/1 -> Add/2
  Gain2/1 -> Add/1
  T1/1 -> Add2/1
  Tk/1 -> Add2/2
  Add2/1 -> Gain2/1, Gain3/1

== system zhengji/GT2/PT/turbine_TN/K1 ==
  note: Cp
  note: Cv
  T1 : Inport
  Add : Sum
  Add1 : Sum
  Add2 : Sum  Inputs=+-
  Constant : Constant  Value=0.9956
  Constant1 : Constant  Value=0.7088
  Divide1 : Product  Inputs=*/
  Gain2 : Gain  Gain=0.000093
  Gain3 : Gain  Gain=0.000093
  Tk : Constant  Value=273.15
  K : Outport
  Cp : Outport  Port=2
  wires:
  Add/1 -> Divide1/1, Cp/1
  Constant/1 -> Add/2
  Gain2/1 -> Add/1
  T1/1 -> Add2/1
  Tk/1 -> Add2/2
  Add2/1 -> Gain2/1, Gain3/1
  Divide1/1 -> K/1
  Add1/1 -> Divide1/2
  Constant1/1 -> Add1/2
  Gain3/1 -> Add1/1
